simulink model "test_diode"  (R2013a)
settings: Solver=ode15s  StartTime=0.0  StopTime=0.1  MaxStep=0.001  RelTol=1e-3
libraries: fl_lib x9, nesl_utility x4
settings Model: Creator=Administrator  LastModifiedBy=Administrator
settings DebuggingCC: SolverPrmCheckMsg=none

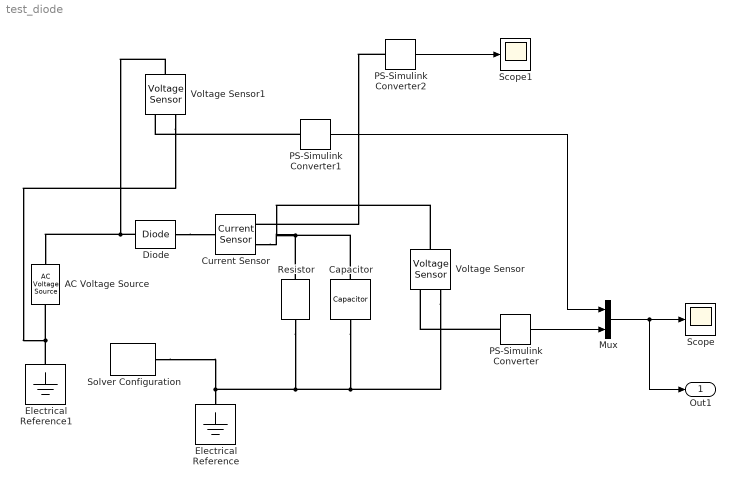
== system test_diode ==
  AC Voltage Source : fl_lib/Electrical/Electrical Sources/AC Voltage Source  amp=150 V  shift=0 deg  frequency=60 Hz  omega=0 rad/s  i_Log=off  v_Log=off  LocalVarNames=|i|v  LocalVarDescs=|i|v  LocalVarLogging=[0 0]
  Capacitor : fl_lib/Electrical/Electrical Elements/Capacitor  c=10e-6 F  v0=0 V  r=1e-6 Ohm  g=0 1/Ohm  i_Log=off  v_Log=off  vc_Log=off  LocalVarNames=|i|v|vc  LocalVarDescs=|i|v|Internal variable for voltage across capacitor term  LocalVarLogging=[0 0 0]
  Current Sensor : fl_lib/Electrical/Electrical Sensors/Current Sensor  i1_Log=off  v1_Log=off  LocalVarNames=|i1|v1  LocalVarDescs=|i1|v1  LocalVarLogging=[0 0]
  Diode : fl_lib/Electrical/Electrical Elements/Diode  Vf=0.6 V  Ron=0.3 Ohm  Goff=1e-8 1/Ohm  i_Log=off  v_Log=off  LocalVarNames=|i|v  LocalVarDescs=|i|v  LocalVarLogging=[0 0]
  Electrical Reference : fl_lib/Electrical/Electrical Elements/Electrical Reference  i_Log=off  LocalVarNames=|i  LocalVarDescs=|i  LocalVarLogging=0
  Electrical Reference1 : fl_lib/Electrical/Electrical Elements/Electrical Reference  i_Log=off  LocalVarNames=|i  LocalVarDescs=|i  LocalVarLogging=0
  Mux : Mux  Inputs=2
  PS-Simulink Converter : nesl_utility/PS-Simulink Converter  PhysicalDomain=network_engine_domain  SubClassName=ps_output  LeftPortType=input  RightPortType=output  PseudoPeriodic=off  Frequencies=[]  Unit=1  AffineConversion=off
  PS-Simulink Converter1 : nesl_utility/PS-Simulink Converter  PhysicalDomain=network_engine_domain  SubClassName=ps_output  LeftPortType=input  RightPortType=output  PseudoPeriodic=off  Frequencies=[]  Unit=1  AffineConversion=off
  PS-Simulink Converter2 : nesl_utility/PS-Simulink Converter  PhysicalDomain=network_engine_domain  SubClassName=ps_output  LeftPortType=input  RightPortType=output  PseudoPeriodic=off  Frequencies=[]  Unit=1  AffineConversion=off
  Resistor : fl_lib/Electrical/Electrical Elements/Resistor  R=1000 Ohm  i_Log=off  v_Log=off  LocalVarNames=|i|v  LocalVarDescs=|i|v  LocalVarLogging=[0 0]
  Scope : Scope
  Scope1 : Scope
  Solver Configuration : nesl_utility/Solver Configuration  PhysicalDomain=network_engine_domain  SubClassName=solver  LeftPortType=input  RightPortType=generic  Accelerate=off  Tones=[]  Harmonics=[]  SimulateNoise=off  Profile=off  UseLocalSampling=off  EnableSwitchedLinearOptims=on  FrequencyDomain=off  UseCCode=off  UseNewInitialization=off  DoDC=off  ResidualTolerance=1e-09  UseLocalSolver=off  LocalSolverChoice=NE_BACKWARD_EULER_ADVANCER  LocalSolverSampleTime=0.001  DoFixedCost=off  MaxNonlinIter=3  MaxModeIter=2  LinearAlgebra=Sparse  DelaysMemoryBudget=1024
  Voltage Sensor : fl_lib/Electrical/Electrical Sensors/Voltage Sensor  i1_Log=off  v1_Log=off  LocalVarNames=|i1|v1  LocalVarDescs=|i1|v1  LocalVarLogging=[0 0]
  Voltage Sensor1 : fl_lib/Electrical/Electrical Sensors/Voltage Sensor  i1_Log=off  v1_Log=off  LocalVarNames=|i1|v1  LocalVarDescs=|i1|v1  LocalVarLogging=[0 0]
  Out1 : Outport
  wires:
  PS-Simulink Converter/1 -> Mux/2
  Mux/1 -> Out1/1, Scope/1
  PS-Simulink Converter1/1 -> Mux/1
  PS-Simulink Converter2/1 -> Scope1/1
  connections:
  Voltage Sensor/RConn2 -- Capacitor/RConn1 -- Resistor/RConn1 -- Solver Configuration/RConn1 -- Electrical Reference/LConn1
  PS-Simulink Converter/LConn1 -- Voltage Sensor/RConn1
  Electrical Reference1/LConn1 -- Voltage Sensor1/RConn2 -- AC Voltage Source/RConn1
  PS-Simulink Converter1/LConn1 -- Voltage Sensor1/RConn1
  Resistor/LConn1 -- Current Sensor/RConn2 -- Voltage Sensor/LConn1 -- Capacitor/LConn1
  Diode/LConn1 -- AC Voltage Source/LConn1 -- Voltage Sensor1/LConn1
  Diode/RConn1 -- Current Sensor/LConn1
  PS-Simulink Converter2/LConn1 -- Current Sensor/RConn1
